simulink model "simulink_lab_7_pulse_modulation"  (R2022b)
settings: Solver=VariableStepAuto  StartTime=0.0  StopTime=10.0  RelTol=1e-3
libraries: simulink x1, spsMonostableLib x1, spsSawtoothGeneratorLib x1
settings Model: Creator=14200  LastModifiedBy=14200

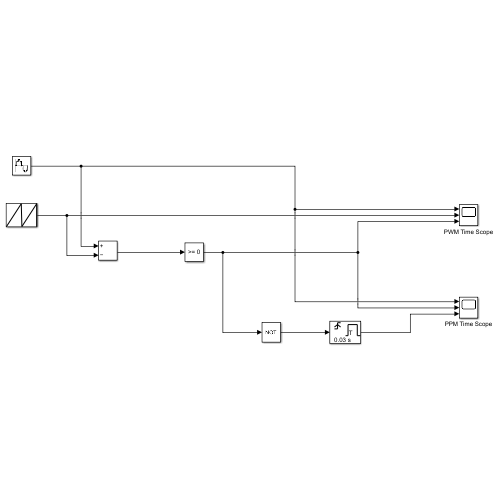
[thumbnail: Simulink's stored preview of the top-level diagram]
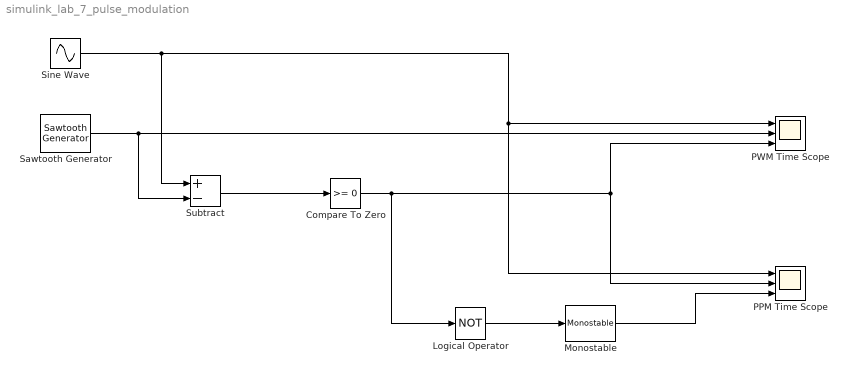
== system simulink_lab_7_pulse_modulation ==
  Compare To Zero : simulink/Logic and Bit Operations/Compare To Zero  relop=>=  OutDataTypeStr=boolean
  Logical Operator : Logic  Operator=NOT  AllPortsSameDT=off  OutDataTypeStr=boolean
  Monostable : spsMonostableLib/Monostable  EdgeDetect=Rising  PulseDuration=0.03  ic=0  Ts=0
      settings: LibrarySourceBlock=sps_lib/Control/Monostable
  PPM Time Scope : Scope  NumInputPorts=3
  PWM Time Scope : Scope  NumInputPorts=3
  Sawtooth Generator : spsSawtoothGeneratorLib/Sawtooth Generator  Freq=1  Phase=0  Ts=0
  Sine Wave : Sin  Frequency=5  SampleTime=0.001
  Subtract : Sum  Inputs=+-
  wires:
  Sine Wave/1 -> Subtract/1, PPM Time Scope/1, PWM Time Scope/1
  Subtract/1 -> Compare To Zero/1
  Sawtooth Generator/1 -> Subtract/2, PWM Time Scope/2
  Logical Operator/1 -> Monostable/1
  Monostable/1 -> PPM Time Scope/3
  Compare To Zero/1 -> Logical Operator/1, PPM Time Scope/2, PWM Time Scope/3
